simulink subsystem "DCLoad"  (R2022a)
settings: Solver=VariableStepAuto  StartTime=0.0  StopTime=10.0  RelTol=1e-3
undefined symbols (not defined in the file): Neg, Pos
libraries: fl_lib x4, nesl_utility x4
settings Model: Creator=mmarq  LastModifiedBy=mmarq

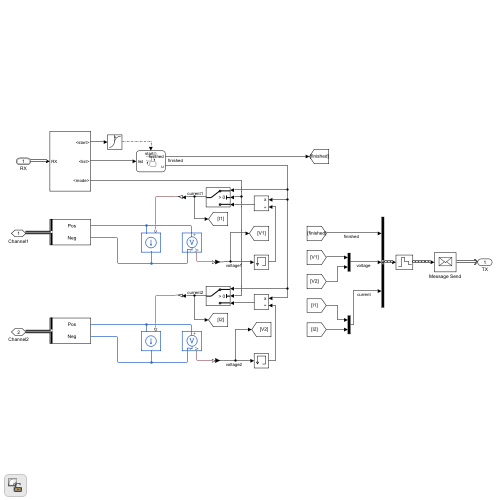
[thumbnail: Simulink's stored preview of the top-level diagram]
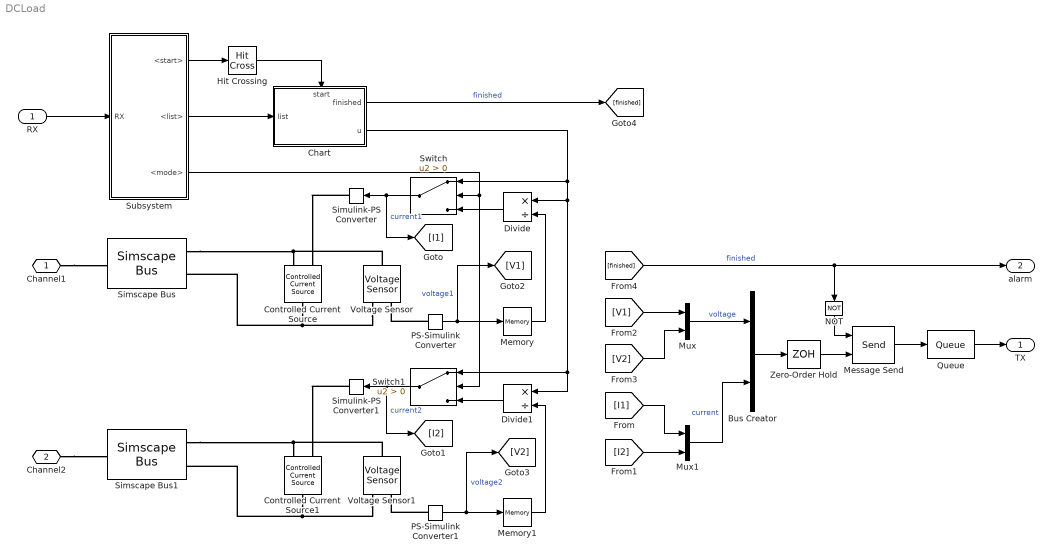
== system DCLoad ==
  RX : Inport  OutputPortMessageModes=m  OutDataTypeStr=Bus: DCLCmd
  Bus Creator : BusCreator  Inputs=2  OutDataTypeStr=Bus: DCLData  NonVirtualBus=on
  Chart : Stateflow chart  TreatAsAtomicUnit=on
      settings: PortSchema="{\"entries\":[{\"content\":{\"sides\":[{\"content\":{\"connectorIds\":[\"In1\"]},\"type\":\"ConnectorPlacement.EquallySpacedRectSide\",\"uuid\":\"4ed828f0-1ac9-4dcc-9380-eef59d4566e8\"},{\"content\":{\"connectorIds\":[\"Out1\",\"Out2\"],\"side\":\"RIGHT\"},\"type\":\"ConnectorPlacement.EquallySpacedRectSide\",\"uuid\":\"89d19431-af69-4c25-9773-8ef87ef26c35\"},{\"content\":{\"connectorIds\":[\"In2\"],\"side\":\"TOP\"},\"type\":\"ConnectorPlacement.EquallySpacedRectSide\",\"uuid\":\"16b2249e-20d7-4791-ad8a-e9d093ae3788\"}]},\"type\":\"ConnectorPlacement.EquallySpacedConnector\",\"uuid\":\"4997d404-275d-4b55-9693-2b863566ce67\"}],\"packageUris\":[\"http://schema.mathworks.com/mf0/Connector/R2020b\"],\"version\":\"1.0\"}"
  Controlled Current Source : fl_lib/Electrical/Electrical Sources/Controlled Current Source
      settings: SourceProductBaseCode=PW,SS,VE
  Controlled Current Source1 : fl_lib/Electrical/Electrical Sources/Controlled Current Source
      settings: SourceProductBaseCode=PW,SS,VE
  Divide : Product  Inputs=*/
  Divide1 : Product  Inputs=*/
  Hit Crossing : HitCross  HitCrossingDirection=rising
  Memory : Memory
  Memory1 : Memory
  Message Send : Send  OutputPortMessageModes=m  ShowEnablePort=on
      settings: InputPortMap=e0,u1
  Mux : Mux  Inputs=2
  Mux1 : Mux  Inputs=2
  NOT : Logic  Operator=NOT  IconShape=distinctive  AllPortsSameDT=off  OutDataTypeStr=boolean
  PS-Simulink Converter : nesl_utility/PS-Simulink Converter  PhysicalDomain=network_engine_domain  SubClassName=ps_output  LeftPortType=input  RightPortType=output  PseudoPeriodic=off  Frequencies=[]  VectorFormat=inherit  Unit=inherit  AffineConversion=off
      settings: SourceProductBaseCode=SS,PW,VE
  PS-Simulink Converter1 : nesl_utility/PS-Simulink Converter  PhysicalDomain=network_engine_domain  SubClassName=ps_output  LeftPortType=input  RightPortType=output  PseudoPeriodic=off  Frequencies=[]  VectorFormat=inherit  Unit=inherit  AffineConversion=off
      settings: SourceProductBaseCode=SS,PW,VE
  Queue : Queue  InputPortMessageModes=m  OutputPortMessageModes=m  OverwriteOldest=on  Capacity=5000000  QueueType=LIFO
  Simscape Bus : SimscapeBus  HierarchyStrings=Pos;Neg
  Simscape Bus1 : SimscapeBus  HierarchyStrings=Pos;Neg
  Simulink-PS Converter : nesl_utility/Simulink-PS Converter  PhysicalDomain=network_engine_domain  SubClassName=ps_input  LeftPortType=input  RightPortType=output  PseudoPeriodic=off  Frequencies=[]  NoiseDistribution=none  NoiseParameters=[]  Unit=1  AffineConversion=off  FilteringAndDerivatives=provide  SimscapeFilterOrder=1  InputFilterTimeConstant=0.001  UdotUserProvided=0
      settings: SourceProductBaseCode=SS,PW,VE
  Simulink-PS Converter1 : nesl_utility/Simulink-PS Converter  PhysicalDomain=network_engine_domain  SubClassName=ps_input  LeftPortType=input  RightPortType=output  PseudoPeriodic=off  Frequencies=[]  NoiseDistribution=none  NoiseParameters=[]  Unit=1  AffineConversion=off  FilteringAndDerivatives=provide  SimscapeFilterOrder=1  InputFilterTimeConstant=0.001  UdotUserProvided=0
      settings: SourceProductBaseCode=SS,PW,VE
  Subsystem : Subsystem
  Switch : Switch  Criteria=u2 > Threshold  SaturateOnIntegerOverflow=off  InputSameDT=off
  Switch1 : Switch  Criteria=u2 > Threshold  SaturateOnIntegerOverflow=off  InputSameDT=off
  Voltage Sensor : fl_lib/Electrical/Electrical Sensors/Voltage Sensor
      settings: SourceProductBaseCode=PW,SS,VE
  Voltage Sensor1 : fl_lib/Electrical/Electrical Sensors/Voltage Sensor
      settings: SourceProductBaseCode=PW,SS,VE
  Zero-Order Hold : ZeroOrderHold  SampleTime=1e-3
  Channel1 : PMIOPort  Side=Left
  Channel2 : PMIOPort  Port=2  Side=Left
  TX : Outport  InputPortMessageModes=m  OutDataTypeStr=Bus: DCLData
  alarm : Outport  Port=2
  wires:
  Subsystem/2(<list>) -> Chart/1(list)
  Chart/2(u) -> Switch/1, Divide1/1, Switch1/1, Divide/1
  Hit Crossing/1 -> Chart/2(start)
  PS-Simulink Converter/1 -> Memory/1, [V1]  "voltage1"
  Divide1/1 -> Switch1/3
  [I1] -> Mux1/1
  [V2] -> Mux/2
  Subsystem/3(<mode>) -> Switch/2, Switch1/2
  Switch1/1 -> Simulink-PS Converter1/1, [I2]  "current2"
  [finished] -> alarm/1, NOT/1  "finished"
  [I2] -> Mux1/2
  Mux1/1 -> Bus Creator/2  "current"
  Bus Creator/1 -> Zero-Order Hold/1
  RX/1 -> Subsystem/1(RX)
  Memory1/1 -> Divide1/2
  PS-Simulink Converter1/1 -> Memory1/1, [V2]  "voltage2"
  Subsystem/1(<start>) -> Hit Crossing/1
  Divide/1 -> Switch/3
  Chart/1(finished) -> [finished]  "finished"
  Memory/1 -> Divide/2
  Switch/1 -> [I1], Simulink-PS Converter/1  "current1"
  Mux/1 -> Bus Creator/1  "voltage"
  [V1] -> Mux/1
  Zero-Order Hold/1 -> Message Send/2
  NOT/1 -> Message Send/1
  Message Send/1 -> Queue/1
  Queue/1 -> TX/1
  connections:
  Controlled Current Source1/LConn1 -- Voltage Sensor1/RConn2 -- Simscape Bus1/LConn2
  Controlled Current Source/LConn1 -- Voltage Sensor/RConn2 -- Simscape Bus/LConn2
  Controlled Current Source/RConn2 -- Voltage Sensor/LConn1 -- Simscape Bus/LConn1
  Controlled Current Source1/RConn2 -- Voltage Sensor1/LConn1 -- Simscape Bus1/LConn1
  PS-Simulink Converter1/LConn1 -- Voltage Sensor1/RConn1
  PS-Simulink Converter/LConn1 -- Voltage Sensor/RConn1
  Simulink-PS Converter1/RConn1 -- Controlled Current Source1/RConn1
  Channel2/RConn1 -- Simscape Bus1/RConn1
  Channel1/RConn1 -- Simscape Bus/RConn1
  Simulink-PS Converter/RConn1 -- Controlled Current Source/RConn1

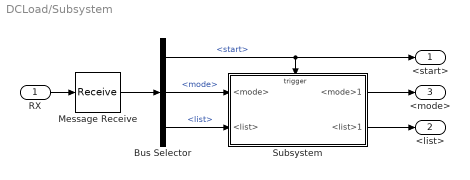
== system DCLoad/Subsystem ==
  RX : Inport  OutDataTypeStr=Bus: DCLCmd
  Bus Selector : BusSelector  OutputSignals=start,mode,list
  Message Receive : Receive  InputPortMessageModes=m  UseInternalQueue=off  QueueOverwriting=on  QueueLength=1  ValueSourceWhenQueueIsEmpty=Use initial value
  Subsystem : Subsystem
  <start> : Outport
  <list> : Outport  Port=2
  <mode> : Outport  Port=3
  wires:
  Subsystem/2(<list>1) -> <list>/1
  Subsystem/1(<mode>1) -> <mode>/1
  Bus Selector/3 -> Subsystem/2(<list>)  "<list>"
  Bus Selector/2 -> Subsystem/1(<mode>)  "<mode>"
  Bus Selector/1 -> Subsystem/Trigger, <start>/1  "<start>"
  RX/1 -> Message Receive/1
  Message Receive/1 -> Bus Selector/1

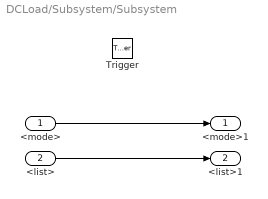
== system DCLoad/Subsystem/Subsystem ==
  <mode> : Inport
  <list> : Inport  Port=2
  Trigger : TriggerPort  VariantControl=(inherit)  PortDimensions=1
  <mode>1 : Outport
  <list>1 : Outport  Port=2
  wires:
  <mode>/1 -> <mode>1/1
  <list>/1 -> <list>1/1

== stateflow chart DCLoad/Chart ==
  settings: sampleTime=0.001  executeAtInitialization=1
  state Idle
    idx = 1;
    u = 0;
  state setOutput
    u=values(idx,1);
  state Next
  Next -> setOutput [order 1] : [idx<100]{idx=idx+1;}
  (default) -> Idle
  Idle -> setOutput : [start==1]{values=list;}
  setOutput -> Next : [after(values(idx,2),sec)]
  Next -> Idle [order 2] : {finished=1;}
  data: finished output; list input; u output; idx local; values local; start input
